simulink model "control_MI_dspic"  (R2018a)
settings: Solver=FixedStepAuto  StartTime=0.0  StopTime=4  FixedStep=Ts  RelTol=1e-5  EnableMultiTasking=on
PreLoadFcn:
  | inicio
InitFcn:
  | mex control_MI_dspic_main.c
values from neighbouring files (symbols this model uses):
  a = ((Llr+Lm).^2.*Rs + Lm.^2.*Rr) ./ (b.*(Llr+Lm))    [param_MI_LV.m]    (also in param_MI_VEU.m)
  A_s = 1.12    [param_veu.m]
  A_v = 1.4    [param_veu.m]
  B = 0.005752    [param_MI_LV.m]    (also in param_veu.m = 1.02)
  b = (Lls+Lm).*(Llr+Lm)-Lm.^2    [param_MI_LV.m]    (also in param_MI_VEU.m)
  B_s = (K_s/d_s)^(1/n_s)    (= 40.3936451136)    [param_veu.m]
  C = 0.68    [param_veu.m]
  C_d = 0.5    [param_veu.m]
  C_r = 0    [param_veu.m]
  C_s = 0.625    [param_veu.m]
  D_s = 1    [param_veu.m]
  eta_t = 0.9    [param_veu.m]
  g = 9.81    [param_veu.m]
  H = 0.47    [param_veu.m]
  H_a = H    (= 0.47)    [param_veu.m]
  J_m = 0.02    [param_veu.m]
  J_t = 0    [param_veu.m]
  J_wf = J_wr    (= 1.95)    [param_veu.m]
  J_wr = 1.95    [param_veu.m]
  L = 1.7    [param_veu.m]
  Lm = 0.00266    [param_MI_LV.m]    (also in param_MI_VEU.m = 0.003940447)
  Lr = (Llr + Lm)    (= 0.00277)    [param_MI_LV.m]    (also in param_MI_VEU.m = 0.004120686)
  Ls = (Lls + Lm)    (= 0.00277)    [param_MI_LV.m]    (also in param_MI_VEU.m = 0.004120686)
  m_v = 590    [param_veu.m]
  N_t = 10.3    [param_veu.m]
  P = 4    [param_MI_LV.m]    (also in param_MI_VEU.m)
  R = 0.268    [param_veu.m]
  ro_v = 1.225    [param_veu.m]
  Rr = 0.03471    [param_MI_LV.m]    (also in param_MI_VEU.m = 0.03841)
  Rs = 0.0697    [param_MI_LV.m]    (also in param_MI_VEU.m = 0.0274)
  sigma = (1- Lm^2/(Ls*Lr))    (= 0.0855669026076)    [param_MI_VEU.m]
  sigma_m = 0.005752    [param_veu.m]
  sigma_wf = sigma_wr    (= 0)    [param_veu.m]
  sigma_wr = 0    [param_veu.m]
  tita_w_0 = 0    [param_veu.m]
  Tr = (Llr+Lm)/Rr    (= 0.07980409104)    [param_MI_LV.m]    (also in param_MI_VEU.m = 0.107281593335)
  Ts = .5e-6    (= 5e-07)    [inicio.m]
  Tsc = 0.000054    (= 5.4e-05)    [inicio.m]    (also in param_MI_VEU.m)
  v_a_revancha = 0    [param_veu.m]
  v_x_0 = 00    (= 0)    [param_veu.m]
  w_w_0 = 0    [param_veu.m]
  x_x_0 = 0    [param_veu.m]
undefined symbols (not defined in the file or in its folder): DiscIntNeverNeededParam
libraries: powerlib x25, simulink x11, dspsigops x2, powerlib_meascontrol x1
(part 1 of 2)
settings Model: SimulationMode=accelerator  Creator=gam  LastModifiedBy=facu
settings SolverCC: AutoInsertRateTranBlk=on
settings DataIOCC: LimitDataPoints=on  SaveFormat=Array  SignalLoggingSaveFormat=ModelDataLogs
settings OptimizationCC: EfficientMapNaN2IntZero=off  LifeSpan=inf
settings DebuggingCC: UnderspecifiedInitializationDetection=Classic  MergeDetectMultiDrivingBlocksExec=none  SolverPrmCheckMsg=warning  FcnCallInpInsideContextMsg=warning  StateNameClashWarn=warning  SFUnexpectedBacktrackingDiag=warning  SFNoUnconditionalDefaultTransitionDiag=warning  SFExecutionAtInitializationDiag=none
settings HardwareCC: ProdBitPerPointer=32  ProdBitPerSizeT=32  ProdBitPerPtrDiffT=32  ProdLargestAtomicFloat=None  ProdIntDivRoundTo=Undefined  ProdEndianess=Unspecified  ProdWordSize=32  ProdHWDeviceType=32-bit Generic  TargetBitPerLong=64  TargetBitPerPointer=64  TargetBitPerSizeT=64  TargetBitPerPtrDiffT=64  TargetLongLongMode=on  TargetIntDivRoundTo=Zero  TargetEndianess=LittleEndian  TargetWordSize=64  TargetHWDeviceType=MATLAB Host  ProdEqTarget=off
settings ModelReferenceCC: PropagateSignalLabelsOutOfModel=off
settings CodeAppCC: MaxIdLength=128
settings GRTTargetCC: TargetLangStandard=C89/C90 (ANSI)  CombineOutputUpdateFcns=off  GRTInterface=on
settings ConfigComp: CovMetricSettings=dw  CovHtmlReporting=on  CovSaveCumulativeToWorkspaceVar=on  CovSaveSingleToWorkspaceVar=on  CovExternalEMLEnable=off
settings SimscapeCC: SimscapeNormalizeSystem=off

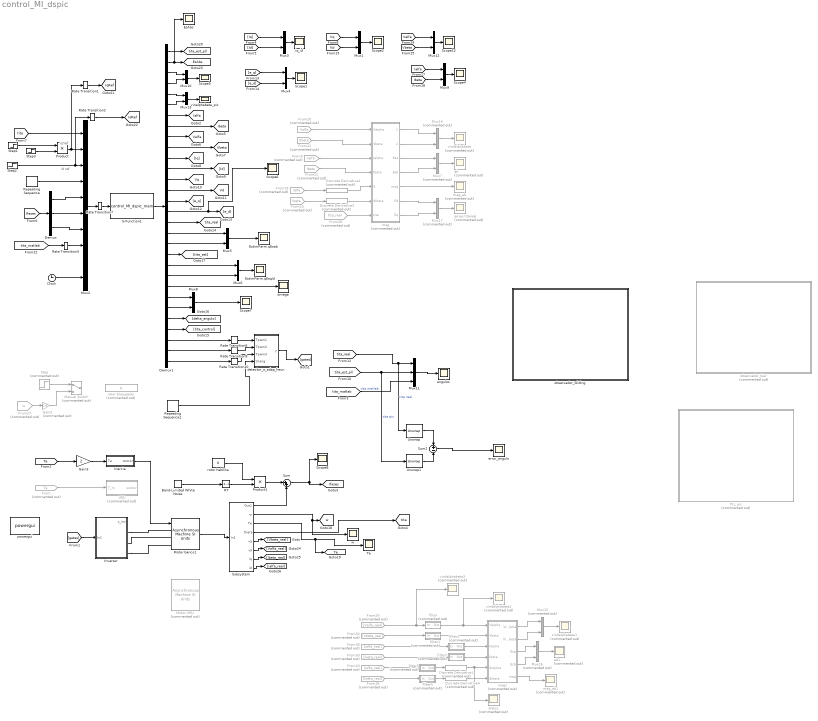
== system control_MI_dspic ==
  note: id ref
  note: iq ref
  Band-Limited White Noise : simulink/Sources/Band-Limited White Noise  Cov=[0.0001]  Ts=Tsc  seed=[23341]
  Clock : Clock
  Demux : Demux  Outputs=3
  Demux1 : Demux  Outputs=30
  Discrete Derivative{1..4} (4 alike) : simulink/Discrete/Discrete Derivative  Commented=on  gainval=1.0  ICPrevScaledInput=0.0  OutMin=[]  OutMax=[]  OutDataType=fixdt(1, 16)  OutScaling=2^-10  DoSatur=off
  EsAbs : Scope
  EstimParm.qEsab : Scope
  EstimParm.qEsq/d : Scope
  From : From  Commented=on  GotoTag=Te  TagVisibility=global
  From11 : From  Commented=on  GotoTag=Ibeta  TagVisibility=global
  From16 : From  Commented=on  GotoTag=Ibeta  TagVisibility=global
  From19 : From  Commented=on  GotoTag=Ialfa  TagVisibility=global
  From20 : From  Commented=on  GotoTag=Valfa  TagVisibility=global
  From21 : From  Commented=on  GotoTag=Vbeta  TagVisibility=global
  From23 : From  Commented=on  GotoTag=ialfa_real
  From26 : From  Commented=on  GotoTag=ibeta_real
  From27 : From  Commented=on  GotoTag=w
  From28 : From  Commented=on  GotoTag=tita_real  TagVisibility=global
  From29 : From  Commented=on  GotoTag=Valfa_real
  From30 : From  Commented=on  GotoTag=ialfa_real
  From32 : From  Commented=on  GotoTag=Vbeta_real
  From33 : From  Commented=on  GotoTag=ibeta_real
  From9 : From  Commented=on  GotoTag=Ialfa  TagVisibility=global
  Gain2 : Gain  Commented=on  Gain=1/9
  Gain3 : Gain  Gain=2
  Inercia : Subsystem
  Inversor : Subsystem
  Manual Switch : ManualSwitch  Commented=on
  Motor VEU : powerlib/Machines/Asynchronous Machine SI Units  Commented=on  RotorType=Squirrel-cage  PresetModel=No  MechanicalLoad=Speed w  ShowDetailedParameters=on  ReferenceFrame=Stationary  Units=SI  MeasurementBus=on  NominalParameters=[3000 48 50]  Stator=[0.0274 0.000180239]  Rotor=[0.03841 0.000180239]  Cage1=[0.4155 0.002066]  Cage2=[0.4168 0.0003495]  Lm=0.003940447  Mechanical=[0.01 0.0000 2]  PolePairs=2  InitialConditions="[ 0,90   0,0,0   0,0,0 ]"  SimulateSaturation=off  Saturation=[9.9249,19.6672,38.0377,51.3988,69.2824,105.1337,152.5532,214.2421,303.1917;230, 322, 414, 460, 506, 552, 598, 644, 690]  LoadFlowParameters=0  TsPowergui=0  TsBlock=-1  IterativeModel=Trapezoidal non iterative  IterativeDiscreteModel=Trapezoidal non iterative  Pmec=1.492e+006
  Motor banco1 : powerlib/Machines/Asynchronous Machine SI Units  RotorType=Squirrel-cage  PresetModel=No  MechanicalLoad=Speed w  ShowDetailedParameters=on  ReferenceFrame=Stationary  Units=SI  MeasurementBus=on  NominalParameters=[750 42 50]  Stator=[0.0697 0.00011]  Rotor=[0.03471 0.00011]  Cage1=[0.4155 0.002066]  Cage2=[0.4168 0.0003495]  Lm=0.00266  Mechanical=[0.01 0.0000 2]  PolePairs=2  InitialConditions="[ 1,0   0,0,0   0,0,0 ]"  SimulateSaturation=off  Saturation=[9.9249,19.6672,38.0377,51.3988,69.2824,105.1337,152.5532,214.2421,303.1917;230, 322, 414, 460, 506, 552, 598, 644, 690]  LoadFlowParameters=0  TsPowergui=0  TsBlock=-1  IterativeModel=Trapezoidal non iterative  IterativeDiscreteModel=Trapezoidal non iterative  Pmec=1.492e+006
  Mux{1,3..6,8..10,12..13} (10 alike) : Mux  Inputs=2
  Mux11 : Mux  Inputs=3
  Mux{7,14..17} (5 alike) : Mux  Commented=on  Inputs=2
  Mux2 : Mux  Inputs=10
  PLL pic : Subsystem  Commented=on
  Product : Product
  Product1 : Product
  RT : RateTransition  OutPortSampleTime=Ts
  Rate Transition1 : RateTransition  OutPortSampleTime=Tsc
  Rate Transition10 : RateTransition  OutPortSampleTimeOpt=Inherit  OutPortSampleTime=Tsc
  Rate Transition2 : RateTransition  OutPortSampleTime=Tsc
  Rate Transition5 : RateTransition
  Rate Transition6 : RateTransition  OutPortSampleTimeOpt=Inherit  OutPortSampleTime=Tsc
  Rate Transition7 : RateTransition  OutPortSampleTime=Tsc
  Rate Transition9 : RateTransition  OutPortSampleTimeOpt=Inherit  OutPortSampleTime=Tsc
  Repeating Sequence : simulink/Sources/Repeating Sequence  rep_seq_t="[0 0.00027  0.00054]"  rep_seq_y="[0     3500        0]"
  Repeating Sequence1 : simulink/Sources/Repeating Sequence  rep_seq_t="[0 0.000027  0.000054]"  rep_seq_y="[0     3500        0]"
  S-Function1 : S-Function  FunctionName=control_MI_dspic_main  SFunctionDeploymentMode=off  EnableBusSupport=off
  Scope{1..2,4..8,12} (8 alike) : Scope
  Step : Step  Commented=on  Time=0.5  After=5  SampleTime=0
  Step1 : Step  Time=0.005  After=6772  SampleTime=0
  Step2 : Step  Time=0.005  After=3823  SampleTime=0
  Step3 : Step  Time=2  Before=1  After=-1  SampleTime=0
  Subsystem : Subsystem
  Sum : Sum  Inputs=|++
  Sum2 : Sum  Inputs=+|-
  Te : Scope
  Unwrap : dspsigops/Unwrap  tol=pi  InputProcessing=Columns as channels (frame based)  running=off
  Unwrap1 : dspsigops/Unwrap  tol=pi  InputProcessing=Columns as channels (frame based)  running=off
  VEU : Subsystem  Commented=on
  ab : Scope  Commented=on
  ab1 : Scope  Commented=on
  angulos : Scope
  detector_a_adap_heun : MATLAB Function  TreatAsAtomicUnit=on
  dialp1 : Scope  Commented=on
  ed eq titareal : Scope  Commented=on
  error_angulo : Scope
  filter : Subsystem  Commented=on  mask(Discrete first-order filter (Low-pass)){T=1/(2*pi*800), Ts=Ts}
      mask prompts: T "Time constant (s):"; Ts "Sample time (s):"
      mask help: This block implements a discrete low-pass filter. To calculate the coefficients, the block discretises a continuous low-pass filter using the Tustin method.
      mask init:
      | num = [ Ts/(2*T + Ts), Ts/(2*T + Ts)];
      | den = [ 1, -(2*T - Ts)/(2*T + Ts)];
  filter1 : Subsystem  Commented=on  mask(Discrete first-order filter (Low-pass)){T=1/(2*pi*800), Ts=Ts}
      mask prompts: T "Time constant (s):"; Ts "Sample time (s):"
      mask help: This block implements a discrete low-pass filter. To calculate the coefficients, the block discretises a continuous low-pass filter using the Tustin method.
      mask init:
      | num = [ Ts/(2*T + Ts), Ts/(2*T + Ts)];
      | den = [ 1, -(2*T - Ts)/(2*T + Ts)];
  filter2 : Subsystem  Commented=on  mask(Discrete first-order filter (Low-pass)){T=1/(2*pi*800), Ts=Ts}
      mask prompts: T "Time constant (s):"; Ts "Sample time (s):"
      mask help: This block implements a discrete low-pass filter. To calculate the coefficients, the block discretises a continuous low-pass filter using the Tustin method.
      mask init:
      | num = [ Ts/(2*T + Ts), Ts/(2*T + Ts)];
      | den = [ 1, -(2*T - Ts)/(2*T + Ts)];
  filter3 : Subsystem  Commented=on  mask(Discrete first-order filter (Low-pass)){T=1/(2*pi*800), Ts=Ts}
      mask prompts: T "Time constant (s):"; Ts "Sample time (s):"
      mask help: This block implements a discrete low-pass filter. To calculate the coefficients, the block discretises a continuous low-pass filter using the Tustin method.
      mask init:
      | num = [ Ts/(2*T + Ts), Ts/(2*T + Ts)];
      | den = [ 1, -(2*T - Ts)/(2*T + Ts)];
  filter4 : Subsystem  Commented=on  mask(Discrete first-order filter (Low-pass)){T=1/(2*pi*300), Ts=Tsc}
      mask prompts: T "Time constant (s):"; Ts "Sample time (s):"
      mask help: This block implements a discrete low-pass filter. To calculate the coefficients, the block discretises a continuous low-pass filter using the Tustin method.
      mask init:
      | num = [ Ts/(2*T + Ts), Ts/(2*T + Ts)];
      | den = [ 1, -(2*T - Ts)/(2*T + Ts)];
  filter5 : Subsystem  Commented=on  mask(Discrete first-order filter (Low-pass)){T=1/(2*pi*300), Ts=Tsc}
      mask prompts: T "Time constant (s):"; Ts "Sample time (s):"
      mask help: This block implements a discrete low-pass filter. To calculate the coefficients, the block discretises a continuous low-pass filter using the Tustin method.
      mask init:
      | num = [ Ts/(2*T + Ts), Ts/(2*T + Ts)];
      | den = [ 1, -(2*T - Ts)/(2*T + Ts)];
  iq_id : Scope
  mag : MATLAB Function  Commented=on  TreatAsAtomicUnit=on
  mag1 : MATLAB Function  Commented=on  TreatAsAtomicUnit=on
  mag_ab : Scope  Commented=on
  mag_ab1 : Scope  Commented=on
  observador_Sliding : Subsystem
  observador_bier : Subsystem  Commented=on
  omega : Scope
  powergui : powerlib/powergui  Priority=1  SimulationMode=Discrete  SampleTime=Ts  frequency=60  Iterations=50  frequencyindice=0  Pbase=100e6  ErrMax=1e-4  UnitsV=kV  UnitsW=MW  buscounter=0  FunctionMessages=off  echomessages=off  EnableUseOfTLC=off  CurrentSourceSwitches=off  DisableSnubberDevices=off  DisableRonSwitches=off  DisableVfSwitches=off  DisplayEquations=off  SolverType=Tustin/Backward Euler (TBE)  Interpol=off  ExternalGateDelay=off  methode=off  Ts=100  x0status=blocks  SPID=off  SwTol=0  HookPort=off  RestoreLinks=warning  ResistiveCurrentMeasurement=off  Frange=[0:2:500]  Ylog=off  Xlog=on  ShowGrid=off  save=off  variable=ZData  structure=0  ZoomFFT=off  StartTime=0.0  cycles=1  DisplayStyle=1  fundamental=60  FreqAxis=off  MaxFrequency=1000  frequencyindicesteady=1  RmsSteady=1  display=off
  rotor bloqueado : Constant  Commented=on  Value=0
  rotor habilita : Constant  Value=0
  vinalphabeta_pic : Scope
  vindalphabeta{,1..3} (4 alike) : Scope  Commented=on
  w : Scope
  tag scope: EsAbs=global, Ialfa=global, Ibeta=global, IdRef=global, Ifases=global, IqRef=global, Te=global, Valfa=global, Vbeta=global, Vd=global, Vq=global, tita=global, tita_est_pll=global, tita_real=global, w=global
  wires:
  S-Function1/1 -> Demux1/1
  [Ifases] -> Demux/1
  Demux/3 -> Mux2/7
  Demux/2 -> Mux2/6
  Demux/1 -> Mux2/5
  Subsystem/3(Te) -> [Te], Te/1
  Mux3/1 -> iq_id/1
  [gates] -> Inversor/1(In1)
  Demux1/7 -> [Ialfa]
  Demux1/8 -> [Ibeta]
  Demux1/9 -> [Valfa]
  Demux1/10 -> [Vbeta]
  Demux1/11 -> [Iq]
  Demux1/12 -> [Id]
  Demux1/13 -> [Vq]
  Demux1/14 -> [Vd]
  Demux1/15 -> [e_q]
  Demux1/16 -> Scope6/1, [e_d]
  Demux1/17 -> [tita_real]
  Demux1/18 -> Mux5/1
  Demux1/19 -> Mux5/2
  [Iq] -> Mux3/1
  [Id] -> Mux3/2
  Demux1/20 -> [tita_est]
  Mux4/1 -> Scope1/1
  [e_q] -> Mux4/1
  [e_d] -> Mux4/2
  Mux1/1 -> Scope2/1
  [Vq] -> Mux1/1
  [Vd] -> Mux1/2
  Demux1/21 -> Mux6/1
  Demux1/22 -> Mux6/2
  Mux6/1 -> EstimParm.qEsq/d/1
  Step2/1 -> Rate Transition2/1, Mux2/3
  Mux12/1 -> Scope12/1
  [Valfa] -> Mux12/1
  [Vbeta] -> Mux12/2
  Subsystem/4(theta) -> [tita]
  Mux9/1 -> Scope4/1
  [Ialfa] -> Mux9/1
  [Ibeta] -> Mux9/2
  Mux5/1 -> EstimParm.qEsab/1
  Demux1/27 -> [tita_control]
  Mux11/1 -> angulos/1
  [tita] -> Mux2/1
  Clock/1 -> Mux2/10
  Demux1/26 -> [delta_angulo]
  Step/1 -> Manual Switch/1
  Subsystem/2(w) -> w/1, [w]
  From27/1 -> Gain2/1
  Gain2/1 -> Manual Switch/2
  Demux1/23 -> omega/1
  Demux1/24 -> Mux8/1
  Demux1/25 -> Mux8/2
  Mux8/1 -> Scope7/1
  [tita_matlab] -> Rate Transition5/1
  Product/1 -> Rate Transition1/1, Mux2/2
  Step1/1 -> Product/1
  Step3/1 -> Product/2
  Mux2/1 -> Rate Transition7/1
  Repeating Sequence/1 -> Mux2/4
  Rate Transition7/1 -> S-Function1/1
  Demux1/28 -> Rate Transition6/1
  Demux1/29 -> Rate Transition9/1
  Demux1/30 -> Rate Transition10/1
  Repeating Sequence1/1 -> detector_a_adap_heun/4(triang)
  Rate Transition6/1 -> detector_a_adap_heun/1(Tpwm1)
  Rate Transition9/1 -> detector_a_adap_heun/2(Tpwm2)
  Rate Transition10/1 -> detector_a_adap_heun/3(Tpwm3)
  detector_a_adap_heun/1(y) -> [gates]
  Rate Transition5/1 -> Mux2/8
  From/1 -> VEU/1(T_m)
  [Te] -> Gain3/1
  Gain3/1 -> Inercia/1(Te)
  Motor banco1/1 -> Subsystem/1(In1)
  Band-Limited White Noise/1 -> RT/1
  Subsystem/1(Out1) -> Sum/2
  Sum/1 -> Scope8/1, [Ifases]
  Inercia/1(wrotor) -> Motor banco1/1
  [tita_matlab] -> Mux11/3  "tita matlab"
  Demux1/1 -> [tita_est_pll]
  [tita_real] -> Unwrap/1, Mux11/1  "tita real"
  [tita_est_pll] -> Unwrap1/1, Mux11/2  "tita pic"
  RT/1 -> Product1/2
  Product1/1 -> Sum/1
  rotor habilita/1 -> Product1/1
  Rate Transition1/1 -> [IqRef]
  Rate Transition2/1 -> [IdRef]
  Demux1/2 -> EsAbs/1, [EsAbs]
  Unwrap/1 -> Sum2/1
  Unwrap1/1 -> Sum2/2
  Sum2/1 -> error_angulo/1
  Mux10/1 -> Scope5/1
  Mux13/1 -> vinalphabeta_pic/1
  Demux1/3 -> Mux10/1
  Demux1/4 -> Mux10/2
  Demux1/5 -> Mux13/1
  Demux1/6 -> Mux13/2
  From9/1 -> mag/3(Ialpha)
  From11/1 -> mag/4(Ibeta)
  From19/1 -> Discrete Derivative2/1
  From16/1 -> Discrete Derivative3/1
  From21/1 -> mag/2(Vbeta)
  From20/1 -> mag/1(Valpha)
  Discrete Derivative3/1 -> mag/6(dIbeta)
  Mux7/1 -> ab/1
  mag/3(Esa) -> Mux7/1
  mag/4(Esb) -> Mux7/2
  mag/5(mag) -> mag_ab/1
  mag/2(VIndbeta) -> Mux14/2
  mag/1(VIndalpha) -> Mux14/1
  Mux14/1 -> vindalphabeta/1
  mag1/1(VIndalpha) -> Mux15/1
  mag1/2(VIndbeta) -> Mux15/2
  mag1/5(mag) -> mag_ab1/1
  mag1/4(Esb) -> Mux16/2
  Discrete Derivative1/1 -> dialp1/1, mag1/5(dIalpha)
  Discrete Derivative4/1 -> mag1/6(dIbeta)
  Mux16/1 -> ab1/1
  mag1/3(Esa) -> Mux16/1
  Mux15/1 -> vindalphabeta1/1
  Subsystem/5(vq) -> [Vbeta_real]
  Subsystem/6(vd) -> [Valfa_real]
  Subsystem/7(iq) -> [ibeta_real]
  Subsystem/8(id) -> [ialfa_real]
  From29/1 -> vindalphabeta3/1, filter/1(In)
  From32/1 -> filter1/1(In)
  From30/1 -> filter3/1(In)
  From33/1 -> filter2/1(In)
  From23/1 -> filter5/1(In)
  From26/1 -> filter4/1(In)
  filter/1(Out) -> vindalphabeta2/1, mag1/1(Valpha)
  filter1/1(Out) -> mag1/2(Vbeta)
  filter2/1(Out) -> mag1/4(Ibeta)
  filter3/1(Out) -> mag1/3(Ialpha)
  filter4/1(Out) -> Discrete Derivative4/1
  filter5/1(Out) -> Discrete Derivative1/1
  From28/1 -> mag/7(tita)
  Mux17/1 -> ed eq titareal/1
  mag/6(Ed) -> Mux17/1
  mag/7(Eq) -> Mux17/2
  Discrete Derivative2/1 -> mag/5(dIalpha)
  connections:
  Inversor/RConn1 -- Motor banco1/LConn1
  Inversor/RConn2 -- Motor banco1/LConn2
  Inversor/RConn3 -- Motor banco1/LConn3

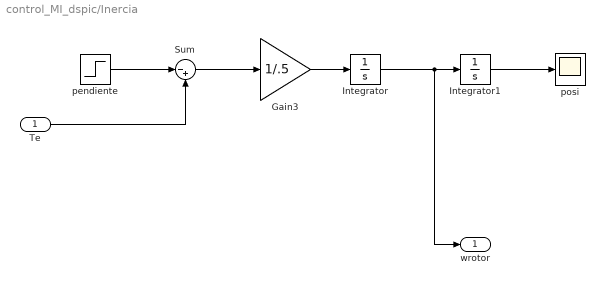
== system control_MI_dspic/Inercia ==
  Te : Inport
  Gain3 : Gain  Gain=1/.5
  Integrator : Integrator
  Integrator1 : Integrator
  Sum : Sum  Inputs=|-+
  pendiente : Step  Time=.5  After=2*0  SampleTime=0
  posi : Scope
  wrotor : Outport
  wires:
  Sum/1 -> Gain3/1
  pendiente/1 -> Sum/1
  Integrator/1 -> wrotor/1, Integrator1/1
  Te/1 -> Sum/2
  Gain3/1 -> Integrator/1
  Integrator1/1 -> posi/1

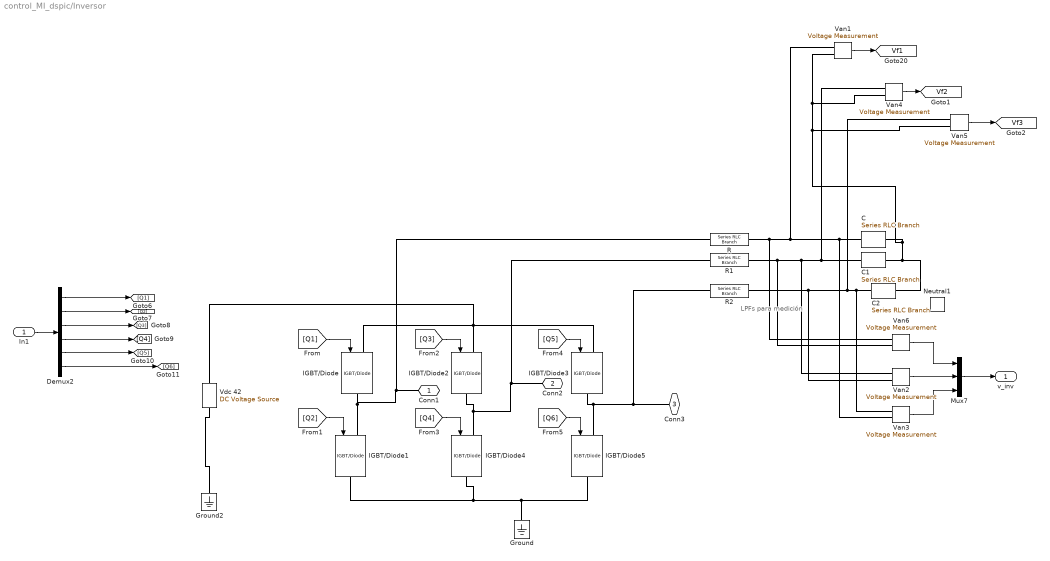
== system control_MI_dspic/Inversor ==
  note: LPFs para medición
  In1 : Inport
  C : powerlib/Elements/Series RLC Branch  LConnTagsString=__new0  RConnTagsString=__new0  BranchType=C  Resistance=10000  Inductance=1e-3  SetiL0=off  InitialCurrent=0  Capacitance=0.1e-6  Setx0=off  InitialVoltage=0  Measurements=Branch voltage and current
  C1 : powerlib/Elements/Series RLC Branch  LConnTagsString=__new0  RConnTagsString=__new0  BranchType=C  Resistance=10000  Inductance=1e-3  SetiL0=off  InitialCurrent=0  Capacitance=0.1e-6  Setx0=off  InitialVoltage=0  Measurements=Branch voltage and current
  C2 : powerlib/Elements/Series RLC Branch  LConnTagsString=__new0  RConnTagsString=__new0  BranchType=C  Resistance=10000  Inductance=1e-3  SetiL0=off  InitialCurrent=0  Capacitance=0.1e-6  Setx0=off  InitialVoltage=0  Measurements=Branch voltage and current
  Demux2 : Demux  Outputs=6
  Ground : powerlib/Elements/Ground  LConnTagsString=a
  Ground2 : powerlib/Elements/Ground  LConnTagsString=a
  IGBT/Diode{,1..5} (6 alike) : powerlib/Power Electronics/IGBT//Diode  Ron=1e-3  Rs=1e5  Cs=inf  Measurements=off
  Mux7 : Mux  Inputs=3
  Neutral1 : powerlib/Elements/Neutral  LConnTagsString=a  NodeNumber=10
      settings: SourceProductName=Simscape Power Systems  SourceProductBaseCode=PS
  R : powerlib/Elements/Series RLC Branch  LConnTagsString=__new0  RConnTagsString=__new0  BranchType=R  Resistance=500  Inductance=1e-3  SetiL0=off  InitialCurrent=0  Capacitance=0.1e-6  Setx0=off  InitialVoltage=0  Measurements=Branch voltage and current
  R1 : powerlib/Elements/Series RLC Branch  LConnTagsString=__new0  RConnTagsString=__new0  BranchType=R  Resistance=500  Inductance=1e-3  SetiL0=off  InitialCurrent=0  Capacitance=0.1e-6  Setx0=off  InitialVoltage=0  Measurements=Branch voltage and current
  R2 : powerlib/Elements/Series RLC Branch  LConnTagsString=__new0  RConnTagsString=__new0  BranchType=R  Resistance=500  Inductance=1e-3  SetiL0=off  InitialCurrent=0  Capacitance=0.1e-6  Setx0=off  InitialVoltage=0  Measurements=Branch voltage and current
  Van{1..6} (6 alike) : powerlib/Measurements/Voltage Measurement  PhasorSimulation=off  OutputType=Complex  PSBequivalent=0
  Vdc 42 : powerlib/Electrical Sources/DC Voltage Source  Amplitude=42  Measurements=None
  Conn1 : PMIOPort  Side=Right
  Conn2 : PMIOPort  Port=2  Side=Right
  Conn3 : PMIOPort  Port=3  Side=Right
  v_inv : Outport
  tag scope: Vf1=global, Vf2=global, Vf3=global
  wires:
  In1/1 -> Demux2/1
  Demux2/4 -> [Q4]
  Demux2/6 -> [Q6]
  Demux2/3 -> [Q3]
  Demux2/1 -> [Q1]
  Demux2/2 -> [Q2]
  Demux2/5 -> [Q5]
  [Q1] -> IGBT/Diode/1
  [Q2] -> IGBT/Diode1/1
  [Q3] -> IGBT/Diode2/1
  [Q4] -> IGBT/Diode4/1
  [Q5] -> IGBT/Diode3/1
  [Q6] -> IGBT/Diode5/1
  Van5/1 -> [Vf3]
  Van2/1 -> Mux7/2
  Van4/1 -> [Vf2]
  Van3/1 -> Mux7/3
  Van1/1 -> [Vf1]
  Van6/1 -> Mux7/1
  Mux7/1 -> v_inv/1
  connections:
  IGBT/Diode/RConn1 -- R/LConn1 -- Conn1/RConn1 -- IGBT/Diode1/LConn1
  IGBT/Diode5/LConn1 -- R2/LConn1 -- Conn3/RConn1 -- IGBT/Diode3/RConn1
  IGBT/Diode2/RConn1 -- R1/LConn1 -- Conn2/RConn1 -- IGBT/Diode4/LConn1
  Vdc 42/LConn1 -- Ground2/LConn1
  Vdc 42/RConn1 -- IGBT/Diode3/LConn1 -- IGBT/Diode2/LConn1 -- IGBT/Diode/LConn1
  IGBT/Diode4/RConn1 -- IGBT/Diode1/RConn1 -- IGBT/Diode5/RConn1 -- Ground/LConn1
  R2/RConn1 -- C2/LConn1 -- Van3/LConn1 -- Van5/LConn1 -- Van2/LConn2
  Van1/LConn2 -- Van4/LConn2 -- C2/RConn1 -- C1/RConn1 -- C/RConn1 -- Van5/LConn2
  C/LConn1 -- R/RConn1 -- Van6/LConn1 -- Van1/LConn1 -- Van3/LConn2
  Van2/LConn1 -- R1/RConn1 -- Van6/LConn2 -- Van4/LConn1 -- C1/LConn1

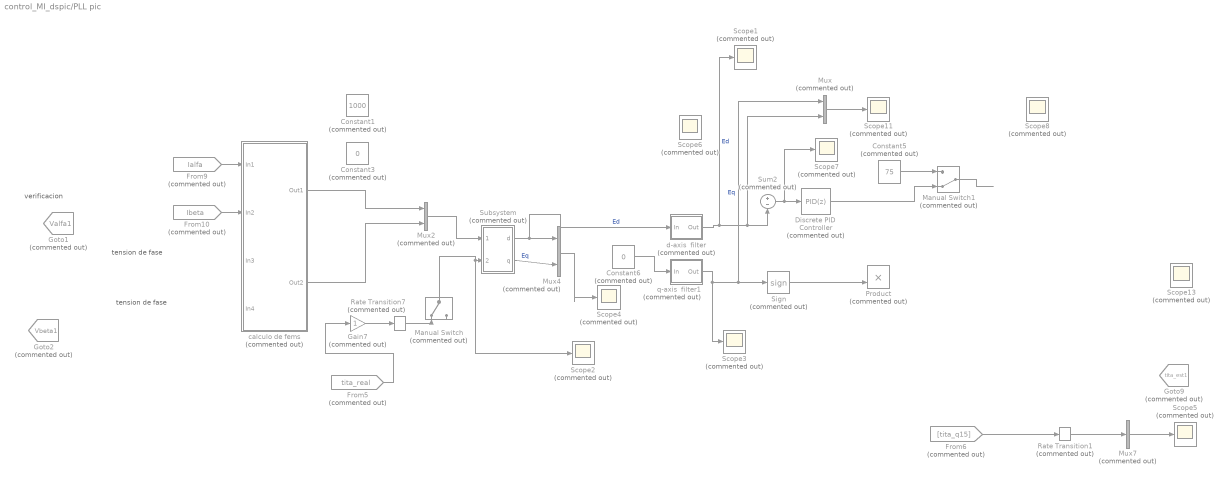
== system control_MI_dspic/PLL pic ==
  note: tension de fase
  note: tension de fase
  note: verificacion
  Constant1 : Constant  Commented=on  Value=1000
  Constant3 : Constant  Commented=on  Value=0
  Constant5 : Constant  Commented=on  Value=75
  Constant6 : Constant  Commented=on  Value=0
  Discrete PID Controller : simulink/Continuous/PID Controller  Commented=on  Controller=PID  TimeDomain=Discrete-time  SampleTime=-1  IntegratorMethod=Forward Euler  FilterMethod=Forward Euler  Form=Parallel  UseFilter=on  ControllerParametersSource=internal  P=500  I=0  D=0  N=100  InitialConditionSource=internal  InitialConditionForIntegrator=0  InitialConditionForFilter=0  ExternalReset=none  LimitOutput=off  UpperSaturationLimit=inf  LowerSaturationLimit=-inf  LinearizeAsGain=off  AntiWindupMode=none  Kb=1  TrackingMode=off  Kt=1  PParamMin=[]  PParamMax=[]  IParamMin=[]  IParamMax=[]  DParamMin=[]  DParamMax=[]  NParamMin=[]  NParamMax=[]  KbParamMin=[]  KbParamMax=[]  KtParamMin=[]  KtParamMax=[]  POutMin=[]  POutMax=[]  IOutMin=[]  IOutMax=[]  DOutMin=[]  DOutMax=[]  NOutMin=[]  NOutMax=[]  KbOutMin=[]  KbOutMax=[]  KtOutMin=[]  KtOutMax=[]  IntegratorOutMin=[]  IntegratorOutMax=[]  FilterOutMin=[]  FilterOutMax=[]  SumOutMin=[]  SumOutMax=[]  SumI1OutMin=[]  SumI1OutMax=[]  SumI2OutMin=[]  SumI2OutMax=[]  SumI3OutMin=[]  SumI3OutMax=[]  SumDOutMin=[]  SumDOutMax=[]  SaturationOutMin=[]  SaturationOutMax=[]  IntegratorContinuousStateAttributes=''  IntegratorStateMustResolveToSignalObject=off  IntegratorRTWStateStorageClass=Auto  FilterContinuousStateAttributes=''  FilterStateMustResolveToSignalObject=off  FilterRTWStateStorageClass=Auto  DifferentiatorICPrevScaledInput=0  DifferentiatorOutMin=[]  DifferentiatorOutMax=[]  FilterDiffOutCoefMin=[]  FilterDiffOutCoefMax=[]  SumDenOutMin=[]  SumDenOutMax=[]  SumNumOutMin=[]  SumNumOutMax=[]  ReciprocalOutMin=[]  ReciprocalOutMax=[]  DivideOutMin=[]  DivideOutMax=[]  TunerSelectOption=Transfer Function Based (PID Tuner App)
  From10 : From  Commented=on  GotoTag=Ibeta  TagVisibility=global
  From5 : From  Commented=on  GotoTag=tita_real  TagVisibility=global
  From6 : From  Commented=on  GotoTag=tita_q15
  From9 : From  Commented=on  GotoTag=Ialfa  TagVisibility=global
  Gain7 : Gain  Commented=on
  Goto1 : Goto  Commented=on  GotoTag=Valfa1  TagVisibility=global
  Goto2 : Goto  Commented=on  GotoTag=Vbeta1  TagVisibility=global
  Goto9 : Goto  Commented=on  GotoTag=tita_est1  TagVisibility=global
  Manual Switch : ManualSwitch  Commented=on
  Manual Switch1 : ManualSwitch  Commented=on  CurrentSetting=0
  Mux : Mux  Commented=on  Inputs=2
  Mux2 : Mux  Commented=on  Inputs=2
  Mux4 : Mux  Commented=on  Inputs=2
  Mux7 : Mux  Commented=on  Inputs=3
  Product : Product  Commented=on
  Rate Transition1 : RateTransition  Commented=on  OutPortSampleTime=0.0001
  Rate Transition7 : RateTransition  Commented=on  OutPortSampleTime=0.0001
  Scope{1..8,11,13} (10 alike) : Scope  Commented=on
  Sign : Signum  Commented=on
  Subsystem : Subsystem  Commented=on
  Sum2 : Sum  Commented=on  Inputs=+-
  calculo de fems : Subsystem  Commented=on
  d-axis  filter : Subsystem  Commented=on  mask(Discrete first-order filter (Low-pass)){T=1/(2*pi*500), Ts=0.0001}
      mask prompts: T "Time constant (s):"; Ts "Sample time (s):"
      mask help: This block implements a discrete low-pass filter. To calculate the coefficients, the block discretises a continuous low-pass filter using the Tustin method.
      mask init:
      | num = [ Ts/(2*T + Ts), Ts/(2*T + Ts)];
      | den = [ 1, -(2*T - Ts)/(2*T + Ts)];
  q-axis  filter1 : Subsystem  Commented=on  mask(Discrete first-order filter (Low-pass)){T=1/(2*pi*500), Ts=0.0001}
      mask prompts: T "Time constant (s):"; Ts "Sample time (s):"
      mask help: This block implements a discrete low-pass filter. To calculate the coefficients, the block discretises a continuous low-pass filter using the Tustin method.
      mask init:
      | num = [ Ts/(2*T + Ts), Ts/(2*T + Ts)];
      | den = [ 1, -(2*T - Ts)/(2*T + Ts)];
  wires:
  ? -> Goto1/1, calculo de fems/3(In3)
  ? -> calculo de fems/4(In4), Goto2/1
  d-axis  filter/1(Out) -> Mux/2, Sum2/2, Scope1/1  "Ed"
  q-axis  filter1/1(Out) -> Scope3/1, Mux/1, Sign/1  "Eq"
  Mux7/1 -> Scope5/1
  Rate Transition1/1 -> Mux7/2
  Manual Switch/1 -> Subsystem/2(theta), Scope2/1
  From6/1 -> Rate Transition1/1
  Gain7/1 -> Rate Transition7/1
  Sum2/1 -> Discrete PID Controller/1, Scope7/1
  Sign/1 -> Product/2
  From5/1 -> Gain7/1
  ? -> Scope13/1, Goto9/1, Manual Switch/2, Mux7/1
  Mux/1 -> Scope11/1
  Rate Transition7/1 -> Manual Switch/1
  From9/1 -> calculo de fems/1(In1)
  From10/1 -> calculo de fems/2(In2)
  calculo de fems/1(Out1) -> Mux2/1
  calculo de fems/2(Out2) -> Mux2/2
  Subsystem/2(q) -> Mux4/2  "Eq"
  Subsystem/1(d) -> d-axis  filter/1(In), Mux4/1  "Ed"
  Constant6/1 -> q-axis  filter1/1(In)
  Mux2/1 -> Subsystem/1(alp bet)
  Mux4/1 -> Scope4/1
  Constant5/1 -> Manual Switch1/1
  Discrete PID Controller/1 -> Manual Switch1/2
  Manual Switch1/1 -> ?

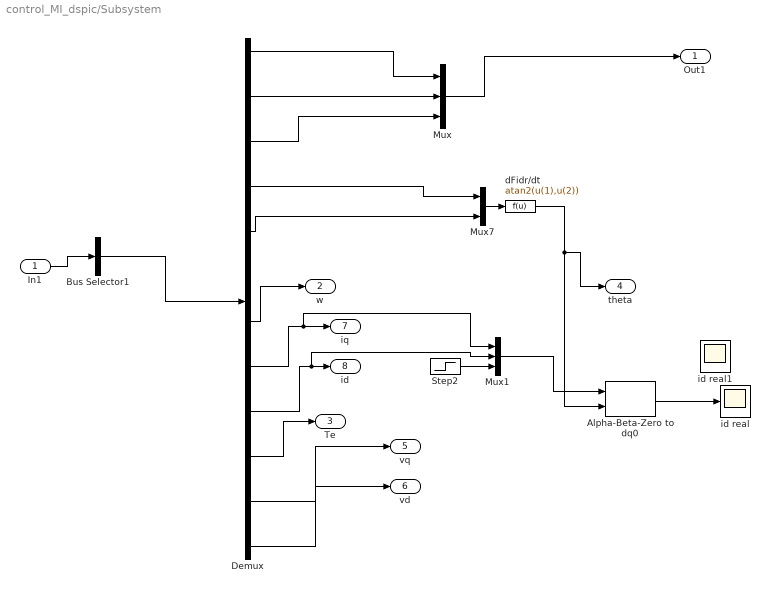
== system control_MI_dspic/Subsystem ==
  In1 : Inport
  Alpha-Beta-Zero to dq0 : powerlib_meascontrol/Transformations/Alpha-Beta-Zero to dq0  Alignment=90 degrees behind phase A axis
      settings: SourceProductName=Simscape Power Systems
  Bus Selector1 : BusSelector  OutputSignals=ias,ibs,ics,phiqr,phidr,theta,w,iqs,ids,Te,vqs,vds  OutputAsBus=on
  Demux : Demux  Outputs=12
  Mux : Mux  Inputs=3
  Mux1 : Mux  Inputs=3
  Mux7 : Mux  Inputs=2
  Step2 : Step  Time=0.005  After=0  SampleTime=0
  dFidr/dt : Fcn  Expr=atan2(u(1),u(2))
  id real : Scope
  id real1 : Scope
  Out1 : Outport
  w : Outport  Port=2
  Te : Outport  Port=3
  theta : Outport  Port=4
  vq : Outport  Port=5
  vd : Outport  Port=6
  iq : Outport  Port=7
  id : Outport  Port=8
  wires:
  In1/1 -> Bus Selector1/1
  Mux7/1 -> dFidr/dt/1
  Mux/1 -> Out1/1
  Bus Selector1/1 -> Demux/1
  Demux/2 -> Mux/2
  Demux/1 -> Mux/1
  Demux/3 -> Mux/3
  Demux/4 -> Mux7/1
  Demux/5 -> Mux7/2
  Demux/7 -> w/1
  dFidr/dt/1 -> Alpha-Beta-Zero to dq0/2, theta/1
  Demux/10 -> Te/1
  Demux/11 -> vq/1
  Demux/12 -> vd/1
  Demux/8 -> Mux1/1, iq/1
  Demux/9 -> Mux1/2, id/1
  Step2/1 -> Mux1/3
  Mux1/1 -> Alpha-Beta-Zero to dq0/1
  Alpha-Beta-Zero to dq0/1 -> id real/1

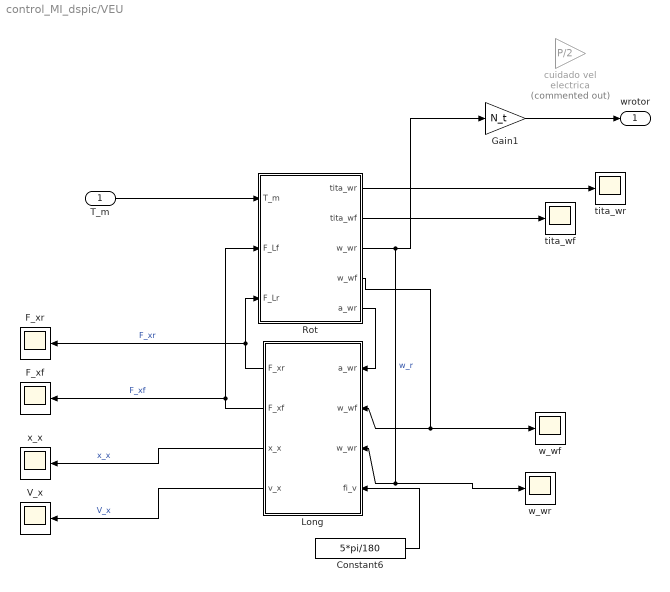
== system control_MI_dspic/VEU ==
  T_m : Inport
  Constant6 : Constant  Value=5*pi/180
  F_xf : Scope
  F_xr : Scope
  Gain1 : Gain  Gain=N_t
  Long : Subsystem
      settings: MinAlgLoopOccurrences=on
  Rot : Subsystem
  V_x : Scope
  cuidado vel electrica : Gain  Commented=on  Gain=P/2
  tita_wf : Scope
  tita_wr : Scope
  w_wf : Scope
  w_wr : Scope
  x_x : Scope
  wrotor : Outport
  wires:
  Long/2(F_xf) -> F_xf/1, Rot/2(F_Lf)  "F_xf"
  Constant6/1 -> Long/4(fi_v)
  Rot/3(w_wr) -> Gain1/1, w_wr/1, Long/3(w_wr)  "w_r"
  Rot/2(tita_wf) -> tita_wf/1
  Long/3(x_x) -> x_x/1  "x_x"
  Rot/5(a_wr) -> Long/1(a_wr)
  Rot/1(tita_wr) -> tita_wr/1
  Long/1(F_xr) -> F_xr/1, Rot/3(F_Lr)  "F_xr"
  Long/4(v_x) -> V_x/1  "V_x"
  Rot/4(w_wf) -> w_wf/1, Long/2(w_wf)
  T_m/1 -> Rot/1(T_m)
  Gain1/1 -> wrotor/1

== system control_MI_dspic/filter ==
  In : Inport
  Discrete Transfer Fcn : DiscreteTransferFcn  Numerator=num  Denominator=den  SampleTime=Ts
  Out : Outport
  wires:
  In/1 -> Discrete Transfer Fcn/1
  Discrete Transfer Fcn/1 -> Out/1

== system control_MI_dspic/filter1 ==
  In : Inport
  Discrete Transfer Fcn : DiscreteTransferFcn  Numerator=num  Denominator=den  SampleTime=Ts
  Out : Outport
  wires:
  Discrete Transfer Fcn/1 -> Out/1
  In/1 -> Discrete Transfer Fcn/1

== system control_MI_dspic/filter2 ==
  In : Inport
  Discrete Transfer Fcn : DiscreteTransferFcn  Numerator=num  Denominator=den  SampleTime=Ts
  Out : Outport
  wires:
  In/1 -> Discrete Transfer Fcn/1
  Discrete Transfer Fcn/1 -> Out/1

== system control_MI_dspic/filter3 ==
  In : Inport
  Discrete Transfer Fcn : DiscreteTransferFcn  Numerator=num  Denominator=den  SampleTime=Ts
  Out : Outport
  wires:
  In/1 -> Discrete Transfer Fcn/1
  Discrete Transfer Fcn/1 -> Out/1

== system control_MI_dspic/filter4 ==
  In : Inport
  Discrete Transfer Fcn : DiscreteTransferFcn  Numerator=num  Denominator=den  SampleTime=Ts
  Out : Outport
  wires:
  Discrete Transfer Fcn/1 -> Out/1
  In/1 -> Discrete Transfer Fcn/1

== system control_MI_dspic/filter5 ==
  In : Inport
  Discrete Transfer Fcn : DiscreteTransferFcn  Numerator=num  Denominator=den  SampleTime=Ts
  Out : Outport
  wires:
  Discrete Transfer Fcn/1 -> Out/1
  In/1 -> Discrete Transfer Fcn/1

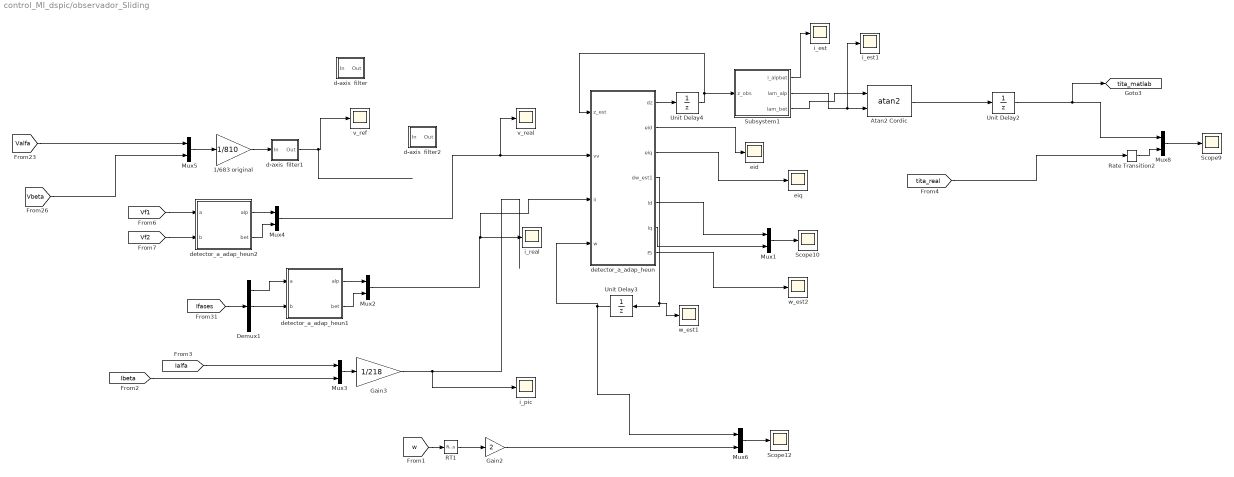
== system control_MI_dspic/observador_Sliding ==
  1/683 original : Gain  Gain=1/810
  Atan2 Cordic : Trigonometry  Operator=atan2  ApproximationMethod=CORDIC
  Demux1 : Demux  Outputs=3
  Gain2 : Gain  Gain=2
  Gain3 : Gain  Gain=1/218
  Mux{1..6,8} (7 alike) : Mux  Inputs=2
  RT1 : RateTransition  OutPortSampleTime=5.4e-05
  Rate Transition2 : RateTransition  OutPortSampleTime=Tsc
  Scope10 : Scope
  Scope12 : Scope
  Scope9 : Scope
  Subsystem1 : Subsystem
  Unit Delay2 : UnitDelay  SampleTime=Tsc
  Unit Delay3 : UnitDelay  SampleTime=Tsc
  Unit Delay4 : UnitDelay  SampleTime=Tsc
  d-axis  filter : Subsystem  mask(Discrete first-order filter (Low-pass)){T=1/(2*pi*800), Ts=Tsc}
      mask prompts: T "Time constant (s):"; Ts "Sample time (s):"
      mask help: This block implements a discrete low-pass filter. To calculate the coefficients, the block discretises a continuous low-pass filter using the Tustin method.
      mask init:
      | num = [ Ts/(2*T + Ts), Ts/(2*T + Ts)];
      | den = [ 1, -(2*T - Ts)/(2*T + Ts)];
  d-axis  filter1 : Subsystem  mask(Discrete first-order filter (Low-pass)){T=1/(2*pi*400), Ts=Tsc}
      mask prompts: T "Time constant (s):"; Ts "Sample time (s):"
      mask help: This block implements a discrete low-pass filter. To calculate the coefficients, the block discretises a continuous low-pass filter using the Tustin method.
      mask init:
      | num = [ Ts/(2*T + Ts), Ts/(2*T + Ts)];
      | den = [ 1, -(2*T - Ts)/(2*T + Ts)];
  d-axis  filter2 : Subsystem  mask(Discrete first-order filter (Low-pass)){T=1/(2*pi*800), Ts=Tsc}
      mask prompts: T "Time constant (s):"; Ts "Sample time (s):"
      mask help: This block implements a discrete low-pass filter. To calculate the coefficients, the block discretises a continuous low-pass filter using the Tustin method.
      mask init:
      | num = [ Ts/(2*T + Ts), Ts/(2*T + Ts)];
      | den = [ 1, -(2*T - Ts)/(2*T + Ts)];
  detector_a_adap_heun : MATLAB Function  TreatAsAtomicUnit=on  SystemSampleTime=Tsc
  detector_a_adap_heun1 : MATLAB Function  TreatAsAtomicUnit=on  SystemSampleTime=Tsc
  detector_a_adap_heun2 : MATLAB Function  TreatAsAtomicUnit=on  SystemSampleTime=Tsc
  eid : Scope
  eiq : Scope
  i_est : Scope
  i_est1 : Scope
  i_pic : Scope
  i_real : Scope
  v_real : Scope
  v_ref : Scope
  w_est1 : Scope
  w_est2 : Scope
  tag scope: tita_matlab=global
  wires:
  Mux3/1 -> Gain3/1
  detector_a_adap_heun/1(dz) -> Unit Delay4/1
  Unit Delay4/1 -> Subsystem1/1(z_obs), detector_a_adap_heun/1(z_est)
  Subsystem1/1(i_alpbet) -> i_est/1
  Mux5/1 -> 1/683 original/1
  detector_a_adap_heun/3(eiq) -> eiq/1
  detector_a_adap_heun/2(eid) -> eid/1
  [w] -> RT1/1
  Mux6/1 -> Scope12/1
  Gain2/1 -> Mux6/2
  Unit Delay3/1 -> detector_a_adap_heun/4(w), Mux6/1
  [tita_real] -> Rate Transition2/1
  Rate Transition2/1 -> Mux8/2
  Mux8/1 -> Scope9/1
  Atan2 Cordic/1 -> Unit Delay2/1
  Subsystem1/3(lam_bet) -> Atan2 Cordic/1
  [Valfa] -> Mux5/1
  [Vbeta] -> Mux5/2
  [Ialfa] -> Mux3/1
  [Ibeta] -> Mux3/2
  detector_a_adap_heun/4(dw_est1) -> w_est1/1, Unit Delay3/1
  detector_a_adap_heun/5(ld) -> Mux1/1
  detector_a_adap_heun/6(lq) -> Mux1/2
  Mux1/1 -> Scope10/1
  Unit Delay2/1 -> [tita_matlab], Mux8/1
  RT1/1 -> Gain2/1
  1/683 original/1 -> d-axis  filter1/1(In)
  Subsystem1/2(lam_alp) -> i_est1/1, Atan2 Cordic/2
  Demux1/2 -> detector_a_adap_heun1/2(b)
  Demux1/1 -> detector_a_adap_heun1/1(a)
  [Ifases] -> Demux1/1
  detector_a_adap_heun1/1(alp) -> Mux2/1
  detector_a_adap_heun1/2(bet) -> Mux2/2
  detector_a_adap_heun2/2(bet) -> Mux4/2
  detector_a_adap_heun2/1(alp) -> Mux4/1
  [Vf1] -> detector_a_adap_heun2/1(a)
  [Vf2] -> detector_a_adap_heun2/2(b)
  Gain3/1 -> i_pic/1
  Mux4/1 -> v_real/1, detector_a_adap_heun/2(vv)
  d-axis  filter1/1(Out) -> v_ref/1
  Mux2/1 -> detector_a_adap_heun/3(ii), i_real/1
  detector_a_adap_heun/7(f5) -> w_est2/1

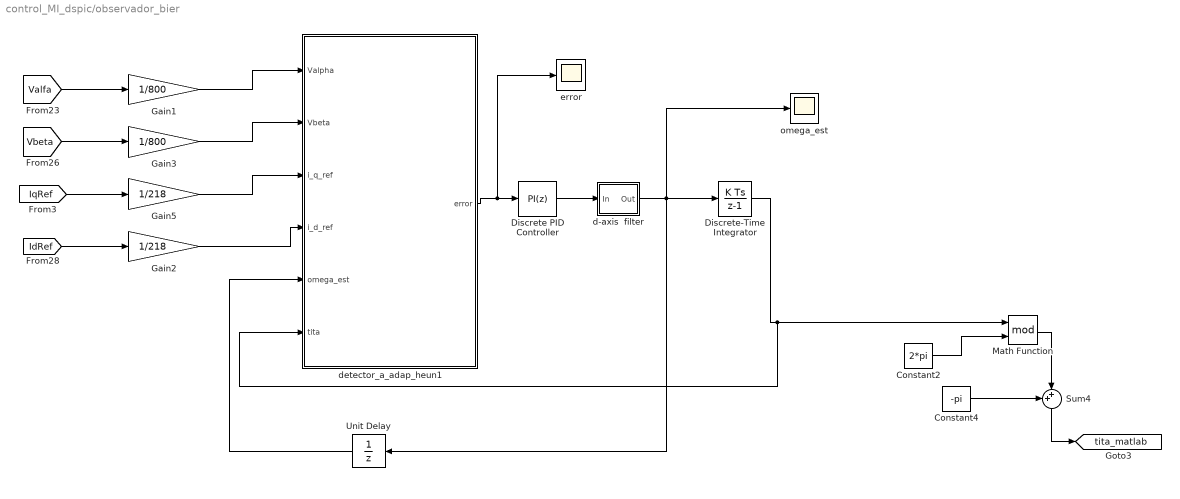
== system control_MI_dspic/observador_bier ==
  Constant2 : Constant  Value=2*pi
  Constant4 : Constant  Value=-pi
  Discrete PID Controller : simulink/Continuous/PID Controller  Controller=PI  TimeDomain=Discrete-time  SampleTime=-1  IntegratorMethod=Forward Euler  FilterMethod=Forward Euler  Form=Parallel  UseFilter=on  ControllerParametersSource=internal  P=10  I=10  D=0  N=100  InitialConditionSource=internal  InitialConditionForIntegrator=0  InitialConditionForFilter=0  ExternalReset=none  LimitOutput=off  UpperSaturationLimit=inf  LowerSaturationLimit=-inf  LinearizeAsGain=off  AntiWindupMode=none  Kb=1  TrackingMode=off  Kt=1  PParamMin=[]  PParamMax=[]  IParamMin=[]  IParamMax=[]  DParamMin=[]  DParamMax=[]  NParamMin=[]  NParamMax=[]  KbParamMin=[]  KbParamMax=[]  KtParamMin=[]  KtParamMax=[]  POutMin=[]  POutMax=[]  IOutMin=[]  IOutMax=[]  DOutMin=[]  DOutMax=[]  NOutMin=[]  NOutMax=[]  KbOutMin=[]  KbOutMax=[]  KtOutMin=[]  KtOutMax=[]  IntegratorOutMin=[]  IntegratorOutMax=[]  FilterOutMin=[]  FilterOutMax=[]  SumOutMin=[]  SumOutMax=[]  SumI1OutMin=[]  SumI1OutMax=[]  SumI2OutMin=[]  SumI2OutMax=[]  SumI3OutMin=[]  SumI3OutMax=[]  SumDOutMin=[]  SumDOutMax=[]  SaturationOutMin=[]  SaturationOutMax=[]  IntegratorContinuousStateAttributes=''  IntegratorStateMustResolveToSignalObject=off  IntegratorRTWStateStorageClass=Auto  FilterContinuousStateAttributes=''  FilterStateMustResolveToSignalObject=off  FilterRTWStateStorageClass=Auto  DifferentiatorICPrevScaledInput=0  DifferentiatorOutMin=[]  DifferentiatorOutMax=[]  FilterDiffOutCoefMin=[]  FilterDiffOutCoefMax=[]  SumDenOutMin=[]  SumDenOutMax=[]  SumNumOutMin=[]  SumNumOutMax=[]  ReciprocalOutMin=[]  ReciprocalOutMax=[]  DivideOutMin=[]  DivideOutMax=[]  TunerSelectOption=Transfer Function Based (PID Tuner App)
  Discrete-Time Integrator : DiscreteIntegrator  InitialCondition=pi  SampleTime=Tsc  ICPrevOutput=DiscIntNeverNeededParam  ICPrevScaledInput=DiscIntNeverNeededParam
  Gain1 : Gain  Gain=1/800
  Gain2 : Gain  Gain=1/218
  Gain3 : Gain  Gain=1/800
  Gain5 : Gain  Gain=1/218
  Math Function : Math  Operator=mod  SaturateOnIntegerOverflow=on
  Sum4 : Sum  Inputs=++|
  Unit Delay : UnitDelay  SampleTime=-1
  d-axis  filter : Subsystem  mask(Discrete first-order filter (Low-pass)){T=1/(2*pi*50), Ts=Tsc}
      mask prompts: T "Time constant (s):"; Ts "Sample time (s):"
      mask help: This block implements a discrete low-pass filter. To calculate the coefficients, the block discretises a continuous low-pass filter using the Tustin method.
      mask init:
      | num = [ Ts/(2*T + Ts), Ts/(2*T + Ts)];
      | den = [ 1, -(2*T - Ts)/(2*T + Ts)];
  detector_a_adap_heun1 : MATLAB Function  TreatAsAtomicUnit=on  SystemSampleTime=Tsc
  error : Scope
  omega_est : Scope
  tag scope: tita_matlab=global
  wires:
  [Valfa] -> Gain1/1
  [Vbeta] -> Gain3/1
  Gain1/1 -> detector_a_adap_heun1/1(Valpha)
  Gain3/1 -> detector_a_adap_heun1/2(Vbeta)
  Gain5/1 -> detector_a_adap_heun1/3(i_q_ref)
  [IqRef] -> Gain5/1
  detector_a_adap_heun1/1(error) -> Discrete PID Controller/1, error/1
  Discrete PID Controller/1 -> d-axis  filter/1(In)
  Gain2/1 -> detector_a_adap_heun1/4(i_d_ref)
  [IdRef] -> Gain2/1
  Discrete-Time Integrator/1 -> detector_a_adap_heun1/6(tita), Math Function/1
  Math Function/1 -> Sum4/2
  Constant2/1 -> Math Function/2
  Constant4/1 -> Sum4/1
  Sum4/1 -> [tita_matlab]
  Unit Delay/1 -> detector_a_adap_heun1/5(omega_est)
  d-axis  filter/1(Out) -> Unit Delay/1, Discrete-Time Integrator/1, omega_est/1

== system control_MI_dspic/PLL pic/Subsystem ==
  alp bet : Inport
  theta : Inport  Port=2
  Mux2 : Mux  Inputs=2
  fd : Fcn  Expr=cos(u(3))*u(1) + sin(u(3))*u(2)
  fq : Fcn  Expr=-sin(u(3))*u(1) + cos(u(3))*u(2)
  d : Outport
  q : Outport  Port=2
  wires:
  theta/1 -> Mux2/2
  Mux2/1 -> fq/1, fd/1
  alp bet/1 -> Mux2/1
  fd/1 -> d/1
  fq/1 -> q/1

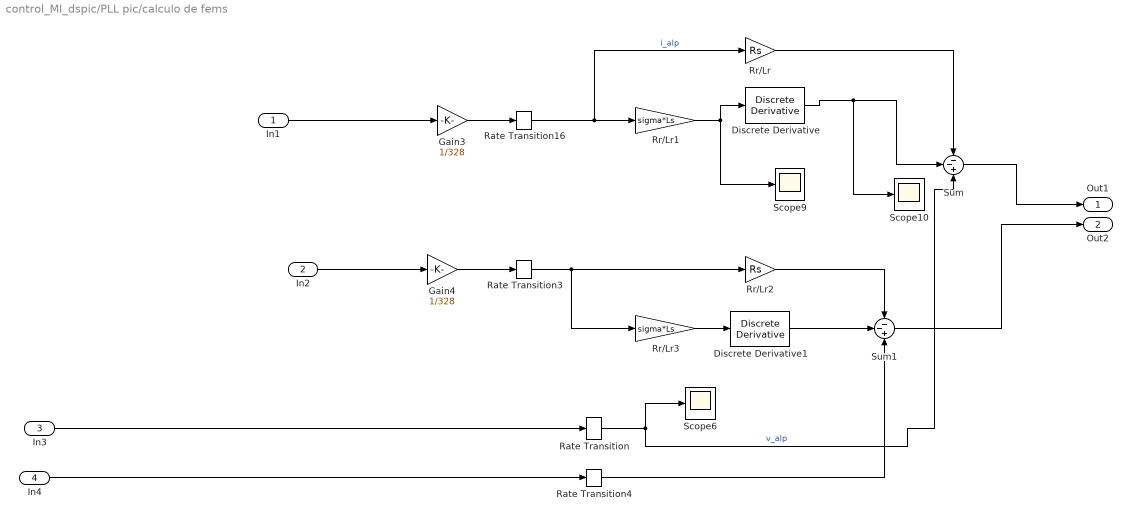
== system control_MI_dspic/PLL pic/calculo de fems ==
  In1 : Inport
  In2 : Inport  Port=2
  In3 : Inport  Port=3
  In4 : Inport  Port=4
  Discrete Derivative : simulink/Discrete/Discrete Derivative  gainval=1  ICPrevScaledInput=0.0  OutMin=[]  OutMax=[]  OutDataType=fixdt(1, 16)  OutScaling=2^-10  DoSatur=off
  Discrete Derivative1 : simulink/Discrete/Discrete Derivative  gainval=1  ICPrevScaledInput=0.0  OutMin=[]  OutMax=[]  OutDataType=fixdt(1, 16)  OutScaling=2^-10  DoSatur=off
  Gain3 : Gain  Gain=1/328
  Gain4 : Gain  Gain=1/328
  Rate Transition{,3..4,16} (4 alike) : RateTransition  OutPortSampleTime=0.0001
  Rr/Lr : Gain  Gain=Rs
  Rr/Lr1 : Gain  Gain=sigma*Ls
  Rr/Lr2 : Gain  Gain=Rs
  Rr/Lr3 : Gain  Gain=sigma*Ls
  Scope10 : Scope
  Scope6 : Scope
  Scope9 : Scope
  Sum : Sum  Inputs=--+
  Sum1 : Sum  Inputs=--+
  Out1 : Outport
  Out2 : Outport  Port=2
  wires:
  Rr/Lr3/1 -> Discrete Derivative1/1
  Rr/Lr1/1 -> Scope9/1, Discrete Derivative/1
  Rr/Lr/1 -> Sum/1
  Discrete Derivative/1 -> Scope10/1, Sum/2
  Rr/Lr2/1 -> Sum1/1
  Rate Transition/1 -> Scope6/1, Sum/3  "v_alp"
  Rate Transition16/1 -> Rr/Lr/1, Rr/Lr1/1  "i_alp"
  Gain4/1 -> Rate Transition3/1
  Sum1/1 -> Out2/1
  Gain3/1 -> Rate Transition16/1
  Rate Transition4/1 -> Sum1/3
  Rate Transition3/1 -> Rr/Lr2/1, Rr/Lr3/1
  Discrete Derivative1/1 -> Sum1/2
  Sum/1 -> Out1/1
  In4/1 -> Rate Transition4/1
  In3/1 -> Rate Transition/1
  In1/1 -> Gain3/1
  In2/1 -> Gain4/1

== system control_MI_dspic/PLL pic/d-axis  filter ==
  In : Inport
  Discrete Transfer Fcn : DiscreteTransferFcn  Numerator=num  Denominator=den  SampleTime=Ts
  Out : Outport
  wires:
  In/1 -> Discrete Transfer Fcn/1
  Discrete Transfer Fcn/1 -> Out/1

== system control_MI_dspic/PLL pic/q-axis  filter1 ==
  In : Inport
  Discrete Transfer Fcn : DiscreteTransferFcn  Numerator=num  Denominator=den  SampleTime=Ts
  Out : Outport
  wires:
  Discrete Transfer Fcn/1 -> Out/1
  In/1 -> Discrete Transfer Fcn/1

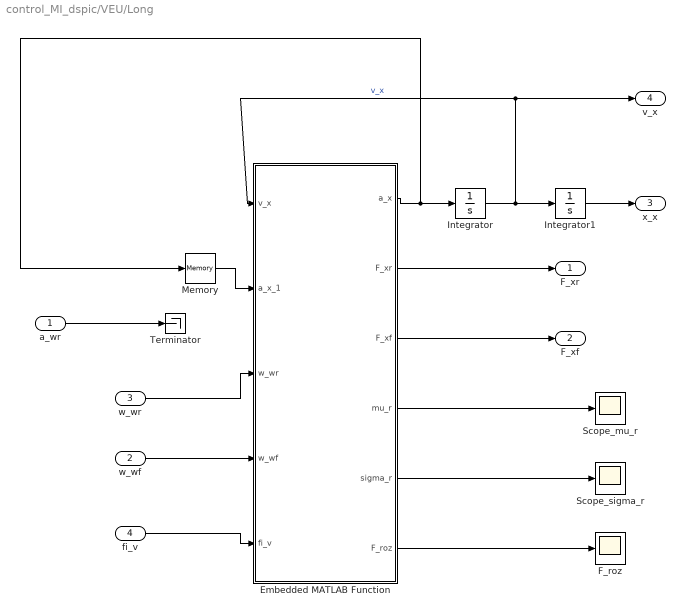
== system control_MI_dspic/VEU/Long ==
  a_wr : Inport
  w_wf : Inport  Port=2  PortDimensions=1
  w_wr : Inport  Port=3
  fi_v : Inport  Port=4  PortDimensions=1
  Embedded MATLAB Function : MATLAB Function
      settings: MinAlgLoopOccurrences=on
  F_roz : Scope
  Integrator : Integrator  InitialCondition=v_x_0
  Integrator1 : Integrator  InitialCondition=x_x_0
  Memory : Memory
  Scope_mu_r : Scope
  Scope_sigma_r : Scope
  Terminator : Terminator
  F_xr : Outport
  F_xf : Outport  Port=2
  x_x : Outport  Port=3
  v_x : Outport  Port=4
  wires:
  Integrator/1 -> Integrator1/1, v_x/1, Embedded MATLAB Function/1(v_x)  "v_x"
  Embedded MATLAB Function/2(F_xr) -> F_xr/1
  w_wf/1 -> Embedded MATLAB Function/4(w_wf)
  Embedded MATLAB Function/3(F_xf) -> F_xf/1
  w_wr/1 -> Embedded MATLAB Function/3(w_wr)
  a_wr/1 -> Terminator/1
  Integrator1/1 -> x_x/1
  Embedded MATLAB Function/1(a_x) -> Memory/1, Integrator/1
  Embedded MATLAB Function/4(mu_r) -> Scope_mu_r/1
  Embedded MATLAB Function/5(sigma_r) -> Scope_sigma_r/1
  fi_v/1 -> Embedded MATLAB Function/5(fi_v)
  Memory/1 -> Embedded MATLAB Function/2(a_x_1)
  Embedded MATLAB Function/6(F_roz) -> F_roz/1

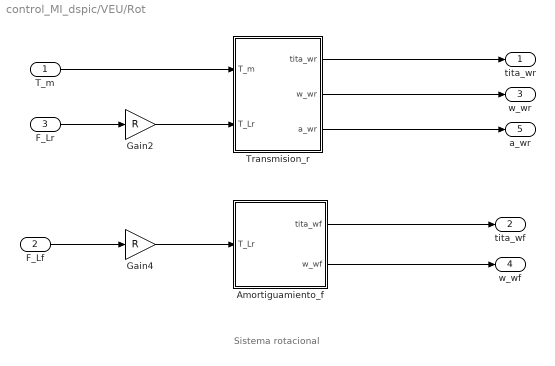
== system control_MI_dspic/VEU/Rot ==
  note: Sistema rotacional
  T_m : Inport
  F_Lf : Inport  Port=2
  F_Lr : Inport  Port=3
  Amortiguamiento_f : Subsystem
  Gain2 : Gain  Gain=R
  Gain4 : Gain  Gain=R
  Transmision_r : Subsystem
  tita_wr : Outport
  tita_wf : Outport  Port=2
  w_wr : Outport  Port=3
  w_wf : Outport  Port=4
  a_wr : Outport  Port=5
  wires:
  T_m/1 -> Transmision_r/1(T_m)
  F_Lr/1 -> Gain2/1
  Gain2/1 -> Transmision_r/2(T_Lr)
  Gain4/1 -> Amortiguamiento_f/1(T_Lr)
  F_Lf/1 -> Gain4/1
  Amortiguamiento_f/1(tita_wf) -> tita_wf/1
  Amortiguamiento_f/2(w_wf) -> w_wf/1
  Transmision_r/1(tita_wr) -> tita_wr/1
  Transmision_r/2(w_wr) -> w_wr/1
  Transmision_r/3(a_wr) -> a_wr/1

== system control_MI_dspic/observador_Sliding/Subsystem1 ==
  z_obs : Inport
  Demux4 : Demux
  Mux : Mux  Inputs=2
  i_alpbet : Outport
  lam_alp : Outport  Port=2
  lam_bet : Outport  Port=3
  wires:
  z_obs/1 -> Demux4/1
  Demux4/2 -> lam_alp/1
  Demux4/1 -> Mux/1
  Demux4/3 -> lam_bet/1
  Mux/1 -> i_alpbet/1
  Demux4/4 -> Mux/2

== system control_MI_dspic/observador_Sliding/d-axis  filter ==
  In : Inport
  Discrete Transfer Fcn : DiscreteTransferFcn  Numerator=num  Denominator=den  SampleTime=Ts
  Out : Outport
  wires:
  In/1 -> Discrete Transfer Fcn/1
  Discrete Transfer Fcn/1 -> Out/1

== system control_MI_dspic/observador_Sliding/d-axis  filter1 ==
  In : Inport
  Discrete Transfer Fcn : DiscreteTransferFcn  Numerator=num  Denominator=den  SampleTime=Ts
  Out : Outport
  wires:
  In/1 -> Discrete Transfer Fcn/1
  Discrete Transfer Fcn/1 -> Out/1

== system control_MI_dspic/observador_Sliding/d-axis  filter2 ==
  In : Inport
  Discrete Transfer Fcn : DiscreteTransferFcn  Numerator=num  Denominator=den  SampleTime=Ts
  Out : Outport
  wires:
  Discrete Transfer Fcn/1 -> Out/1
  In/1 -> Discrete Transfer Fcn/1

== system control_MI_dspic/observador_bier/d-axis  filter ==
  In : Inport
  Discrete Transfer Fcn : DiscreteTransferFcn  Numerator=num  Denominator=den  SampleTime=Ts
  Out : Outport
  wires:
  In/1 -> Discrete Transfer Fcn/1
  Discrete Transfer Fcn/1 -> Out/1

== system control_MI_dspic/VEU/Rot/Amortiguamiento_f ==
  note: Sistema rotacional delantero
  T_Lr : Inport
  Gain : Gain  Gain=1/(J_wf)
  Gain2 : Gain  Gain=sigma_wf
  Integrator : Integrator  InitialCondition=w_w_0
  Integrator1 : Integrator  InitialCondition=tita_w_0
  Sum1 : Sum  Inputs=|+-
  tita_wf : Outport
  w_wf : Outport  Port=2
  wires:
  Gain/1 -> Integrator/1  "a_w"
  Integrator1/1 -> tita_wf/1
  Integrator/1 -> w_wf/1, Gain2/1, Integrator1/1  "w_w"
  Gain2/1 -> Sum1/2
  Sum1/1 -> Gain/1  "a_w"
  T_Lr/1 -> Sum1/1

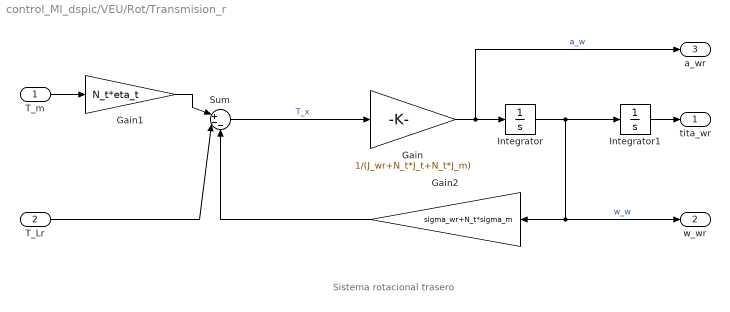
== system control_MI_dspic/VEU/Rot/Transmision_r ==
  note: Sistema rotacional trasero
  T_m : Inport
  T_Lr : Inport  Port=2
  Gain : Gain  Gain=1/(J_wr+N_t*J_t+N_t*J_m)
  Gain1 : Gain  Gain=N_t*eta_t
  Gain2 : Gain  Gain=sigma_wr+N_t*sigma_m
  Integrator : Integrator  InitialCondition=w_w_0
  Integrator1 : Integrator  InitialCondition=tita_w_0
  Sum : Sum  Inputs=|+--
  tita_wr : Outport
  w_wr : Outport  Port=2
  a_wr : Outport  Port=3
  wires:
  T_Lr/1 -> Sum/2
  Gain1/1 -> Sum/1
  T_m/1 -> Gain1/1
  Integrator/1 -> Integrator1/1, Gain2/1, w_wr/1  "w_w"
  Integrator1/1 -> tita_wr/1
  Gain/1 -> Integrator/1, a_wr/1  "a_w"
  Gain2/1 -> Sum/3
  Sum/1 -> Gain/1  "T_x"

== matlab function control_MI_dspic/detector_a_adap_heun ==
  data: Tpwm1 input size=1; Tpwm2 input size=1; Tpwm3 input size=1; y output size=6; triang input size=1
% Facundo Aguilera

% Diseno de filtro para identificar fallas en sensores de corriente
% 2013


function y    = fcn(Tpwm1, Tpwm2, Tpwm3, triang)
     
    DT = 5;
    
    y=zeros(6,1);
    
    if Tpwm1 <= (triang-DT)  
        y(1) = 1;
        y(2) = 0;
    elseif (Tpwm1 >= (triang+DT))   
        y(1) = 0;
        y(2) = 1; 
    else
        y(1) = 0;
        y(2) = 0;
    end

    
    if(Tpwm2 <= (triang-DT))
        y(3) = 1;
        y(4) = 0;
    elseif(Tpwm2 >= (triang+DT))
        y(3) = 0;
        y(4) = 1;
    else           
        y(3) = 0;
        y(4) = 0;
    end

    if(Tpwm3 <= triang-DT) 
        y(5) = 1;
        y(6) = 0;
    
    elseif(Tpwm3 >= (triang+DT))
        y(5) = 0;
        y(6) = 1;
    else 
        y(5) = 0;
        y(6) = 0;
    end
   




end

== matlab function control_MI_dspic/observador_Sliding/detector_a_adap_heun1 ==
  data: alp output size=1; bet output; a input; b input
% Facundo Aguilera

% Diseno de filtro para identificar fallas en sensores de corriente
% 2013


function [alp,bet] = fcn(a, b)

alp = a;
bet = a/sqrt(3)+2*b/sqrt(3);


end

== matlab function control_MI_dspic/observador_Sliding/detector_a_adap_heun ==
  data: z_est input size=4; vv input size=2; ii input size=2; a parameter; dz output size=4; b parameter; Tr parameter; Rs parameter; Ls parameter; Lm parameter; Lr parameter; Rr parameter; Tsc parameter; w input; eid output; eiq output; dw_est1 output; ld output; lq output; f5 output
% Facundo Aguilera

% Diseno de filtro para identificar fallas en sensores de corriente
% 2013


function [dz, eid, eiq, dw_est1,ld,lq,f5] = fcn(z_est, vv, ii,  a, b, Tr, Rs, Ls, Lm, Lr,  Rr, Tsc, w)

% Parametros necesarios
% - Observador
%   k, del
% 
% - Maquina
%   AA, BB

% Entradas



i_d  = ii(1);
i_q  = ii(2);
v_d  = vv(1);
v_q  = vv(2);


i_d_est = z_est(1);
lam_d_est = z_est(2);
lam_q_est = z_est(3);
i_q_est = z_est(4);


% estimador zaki
gama = 30000;


k = 0.001 ;
k1 = 0.01/(Lm/b)*0;
k2 = k*sign(w);

K1 = 200;
K2 = 200;
K3 = (.005 + K1/(Lm/b));
K4 = (.05 + K2/(Lm/b));



% Funciones discontinuas


% == Paso 1
eid = i_d_est - i_d;
eiq = i_q_est - i_q;
%ld = 2/(1+exp(-2*eid))-1;
%lq = 2/(1+exp(-2*eiq))-1;
ld = (eid)./(abs(eid)+50);
lq = (eiq)./(abs(eiq)+50);
v_id = 150*ld;
v_iq = 150*lq;

w_est = w;




f1 = ( Lm/Tr*i_d_est - 1/Tr*lam_d_est - w_est*lam_q_est +( k1*v_id  + k2*v_iq ) );
f2 = ( Lm/Tr*i_q_est - 1/Tr*lam_q_est + w_est*lam_d_est +( -k2*v_id  + k1*v_iq ));
f3 = (-a*i_q_est + Lm/(b*Tr)*lam_q_est - Lm/b*w_est*lam_d_est + Lr/b*v_q - v_iq);
f4 = (-a*i_d_est + Lm/(b*Tr)*lam_d_est + Lm/b*w_est*lam_q_est + Lr/b*v_d - v_id);

f5 = -gama*((ld*lam_q_est - lq*lam_d_est));

lam_d_est1  = lam_d_est + Tsc*f1;
lam_q_est1  = lam_q_est + Tsc*f2;
i_q_est1    = i_q_est   + Tsc*f3;
i_d_est1    = i_d_est   + Tsc*f4;
dw_est1     = w_est     + Tsc*f5;
%dw_est1     = w_est;
% == Paso 2

%eid = i_d_est1 - i_d;
%eiq = i_q_est1 - i_q;
%ld = 2/(1+exp(-2*eid))-1;
%lq = 2/(1+exp(-2*eiq))-1;
%ld = (eid)./(abs(eid)+50);
%lq = (eiq)./(abs(eiq)+50);
%v_id = 50*ld;
%v_iq = 50*lq;



%  f1b = (Lm/Tr*i_d_est1 - 1/Tr*lam_d_est1 - w_est*lam_q_est1 +( k1*v_id  + k2*v_iq ) );
%  f2b = (Lm/Tr*i_q_est1 - 1/Tr*lam_q_est1 + w_est*lam_d_est1 +( -k2*v_id  + k1*v_iq ));
%  f3b = (-a*i_q_est1 + Lm/(b*Tr)*lam_q_est1 - Lm/b*w_est*lam_d_est1 + Lr/b*v_q - K2* v_iq);
%  f4b = (-a*i_d_est1 + Lm/(b*Tr)*lam_d_est1 + Lm/b*w_est*lam_q_est1 + Lr/b*v_d - K1* v_id);
 %f5b = -gama*((ld*lam_q_est1 - lq*lam_d_est1));
% 
% 
%  lam_d_est1 = lam_d_est + Tsc/2*(f1 + f1b );
%  lam_q_est1 = lam_q_est + Tsc/2*(f2 + f2b );
%  i_q_est1   = i_q_est   + Tsc/2*(f3 + f3b ); 
%  i_d_est1   = i_d_est   + Tsc/2*(f4 + f4b );
 %dw_est1    = w_est     + Tsc/2*(f5 + f5b );


%dw_est1= -gama*((ld*lam_q_est1 - lq*lam_d_est1));


dz = [i_d_est1; lam_d_est1; lam_q_est1; i_q_est1];


end

== matlab function control_MI_dspic/mag ==
  data: VIndalpha output; VIndbeta output; Valpha input size=1; Vbeta input size=1; Ialpha input size=1; Ibeta input; dIalpha input; Esa output size=1; Esb output size=1; dIbeta input; mag output; tita input; Ed output; Eq output
% Facundo Aguilera

% Diseno de filtro para identificar fallas en sensores de corriente
% 2013


function [VIndalpha, VIndbeta, Esa, Esb, mag,Ed,Eq]    = fcn(Valpha, Vbeta, Ialpha, Ibeta, dIalpha, dIbeta, tita)
    
    LsDt = 1828*1/18000;
    Rs = 510;

    
    VIndalpha = LsDt * dIalpha/2^7 ;
    VIndbeta  = LsDt * dIbeta/2^7 ;

    Esa		= 	Valpha -	Rs * Ialpha/2^11 - VIndalpha;
    Esb		= 	Vbeta  -	Rs * Ibeta/2^11  - VIndbeta;

    Ed = Esa * cos(tita) + Esb  * sin(tita);
    Eq = Esb * cos(tita) - Esa  * sin(tita);
    
    
    mag = sqrt(Esa^2+Esb^2);

end

== matlab function control_MI_dspic/observador_Sliding/detector_a_adap_heun2 ==
  data: alp output size=1; bet output; a input; b input
% Facundo Aguilera

% Diseno de filtro para identificar fallas en sensores de corriente
% 2013


function [alp,bet] = fcn(a, b)

alp = a;
bet = a/sqrt(3)+2*b/sqrt(3);


end
